simulink model "simula_model"  (R2018a)
settings: Solver=VariableStepAuto  StartTime=0.0  StopTime=Tsim  RelTol=1e-3
values from neighbouring files (symbols this model uses):
  AB = [AB GPC.A^(k-1)*GPC.B]    [model.m]
  Ad = GPC.A^d    [model.m]
  AdD = GPC.A^(d-1)*GPC.D    [model.m]
  d = round(L/Ts)    [model.m]
  delta = [1 -1]    [model.m]
  GPC = gpc_tf2ss_dU(Pz,C,delta,n,nu)    [model.m]
  Kf = K(1,:) * GPC.F    [model.m]
  Kr = K(1,:) * ones(n,1)    [model.m]
  Ts = 0.1    [model.m]
libraries: cstblocks x1
settings Model: Creator=marcus  LastModifiedBy=marcus

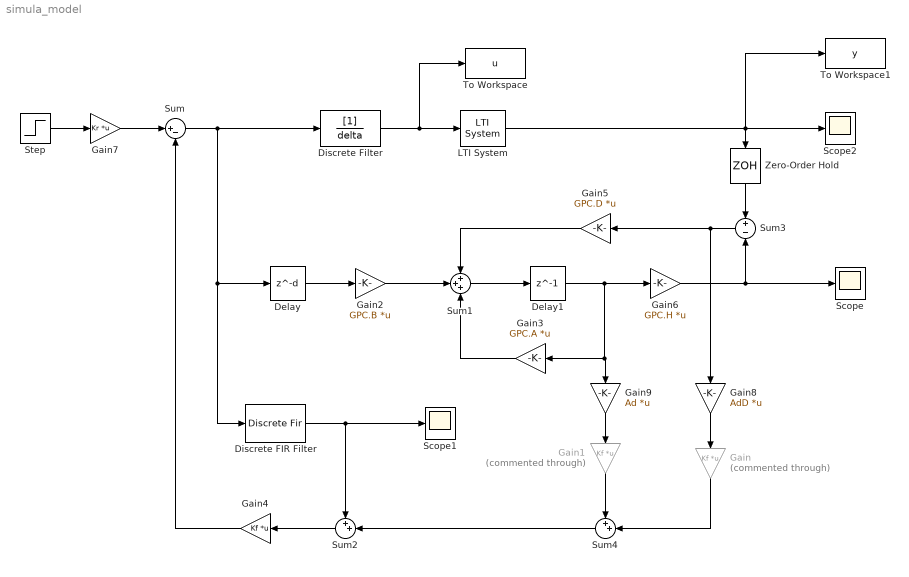
== system simula_model ==
  Delay : Delay  DelayLength=d  SampleTime=Ts
  Delay1 : Delay  DelayLength=1  SampleTime=Ts
  Discrete FIR Filter : DiscreteFir  Coefficients=AB  SampleTime=Ts
  Discrete Filter : DiscreteFilter  Denominator=delta  SampleTime=Ts
  Gain : Gain  Commented=through  Gain=Kf  Multiplication=Matrix(K*u)
  Gain1 : Gain  Commented=through  Gain=Kf  Multiplication=Matrix(K*u)
  Gain2 : Gain  Gain=GPC.B  Multiplication=Matrix(K*u)
  Gain3 : Gain  Gain=GPC.A  Multiplication=Matrix(K*u)
  Gain4 : Gain  Gain=Kf  Multiplication=Matrix(K*u)
  Gain5 : Gain  Gain=GPC.D  Multiplication=Matrix(K*u)
  Gain6 : Gain  Gain=GPC.H  Multiplication=Matrix(K*u)
  Gain7 : Gain  Gain=Kr  Multiplication=Matrix(K*u)
  Gain8 : Gain  Gain=AdD  Multiplication=Matrix(K*u)
  Gain9 : Gain  Gain=Ad  Multiplication=Matrix(K*u)
  LTI System : cstblocks/LTI System  sys=P  IC=[]
  Scope : Scope
  Scope1 : Scope
  Scope2 : Scope
  Step : Step  Time=0  SampleTime=0
  Sum : Sum  Inputs=|+-
  Sum1 : Sum  Inputs=3
  Sum2 : Sum  Inputs=++|
  Sum3 : Sum  Inputs=+-
  Sum4 : Sum  Inputs=++|
  To Workspace : ToWorkspace  VariableName=u  SaveFormat=Timeseries  SampleTime=-1
  To Workspace1 : ToWorkspace  VariableName=y  SaveFormat=Timeseries  SampleTime=-1
  Zero-Order Hold : ZeroOrderHold  SampleTime=Ts
  wires:
  Sum/1 -> Discrete Filter/1, Discrete FIR Filter/1, Delay/1
  Delay/1 -> Gain2/1
  Gain2/1 -> Sum1/2
  Gain3/1 -> Sum1/3
  Step/1 -> Gain7/1
  Sum1/1 -> Delay1/1
  Delay1/1 -> Gain6/1, Gain9/1, Gain3/1
  Gain5/1 -> Sum1/1
  Gain6/1 -> Scope/1, Sum3/2
  Sum3/1 -> Gain8/1, Gain5/1
  Sum2/1 -> Gain4/1
  Gain9/1 -> Gain1/1
  Gain8/1 -> Gain/1
  Sum4/1 -> Sum2/2
  Gain7/1 -> Sum/1
  Discrete Filter/1 -> To Workspace/1, LTI System/1
  LTI System/1 -> To Workspace1/1, Scope2/1, Zero-Order Hold/1
  Zero-Order Hold/1 -> Sum3/1
  Gain1/1 -> Sum4/1
  Gain/1 -> Sum4/2
  Discrete FIR Filter/1 -> Sum2/1, Scope1/1
  Gain4/1 -> Sum/2
